simulink model "seminar2part2"  (R2023a)
settings: Solver=VariableStepAuto  StartTime=0.0  StopTime=1  RelTol=1e-3
libraries: spsDiodeLib x6, spsCurrentMeasurementLib x3, spsRMSLib x3, spsVoltageMeasurementLib x2, spsGroundLib x1, eePowerMeasurement x1, spsParallelRLCBranchLib x1, spsTHDLib x1, spsThreePhaseVIMeasurementLib x1, spsThreePhaseSourceLib x1, spspowerguiLib x1
settings Model: Creator=11094  LastModifiedBy=11094
settings DataIOCC: ReturnWorkspaceOutputs=off

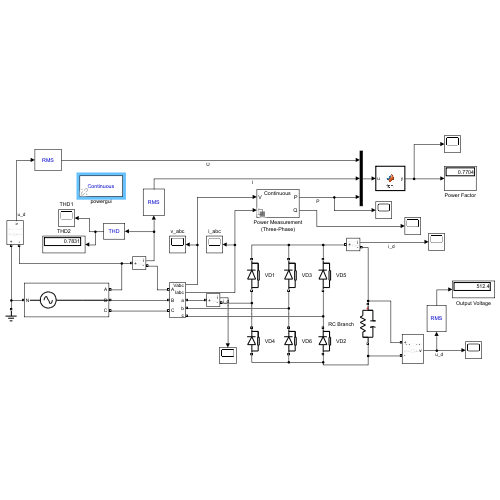
[thumbnail: Simulink's stored preview of the top-level diagram]
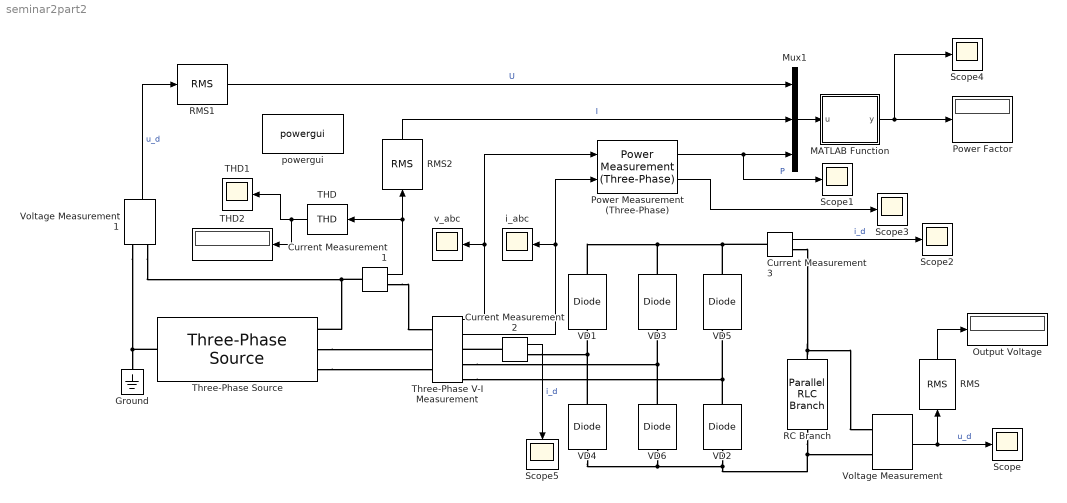
== system seminar2part2 ==
  Current Measurement1 : spsCurrentMeasurementLib/Current Measurement  PhasorSimulation=off  OutputType=Complex  PSBequivalent=0
  Current Measurement2 : spsCurrentMeasurementLib/Current Measurement  PhasorSimulation=off  OutputType=Complex  PSBequivalent=0
  Current Measurement3 : spsCurrentMeasurementLib/Current Measurement  PhasorSimulation=off  OutputType=Complex  PSBequivalent=0
  Ground : spsGroundLib/Ground  LConnTagsString=a
  MATLAB Function : MATLAB Function  TreatAsAtomicUnit=on
  Mux1 : Mux  Inputs=3
  Output Voltage : Display
  Power Factor : Display
  Power Measurement (Three-Phase) : eePowerMeasurement/Power Measurement (Three-Phase)  LabelModeActiveChoice=Continuous  F=50  K=[1]  Seq=Positive  Ts=0
  RC Branch : spsParallelRLCBranchLib/Parallel RLC Branch  LConnTagsString=a  RConnTagsString=__new0  BranchType=RC  Resistance=1  Inductance=1e-3  SetiL0=off  InitialCurrent=0  Capacitance=8e-3  Setx0=off  InitialVoltage=0  Measurements=None
  RMS : spsRMSLib/RMS  TrueRMS=on  Freq=60  RMSInit=120  Ts=0
  RMS1 : spsRMSLib/RMS  TrueRMS=on  Freq=50  RMSInit=120  Ts=0
  RMS2 : spsRMSLib/RMS  TrueRMS=on  Freq=50  RMSInit=120  Ts=0
  Scope{,1..5} (6 alike) : Scope
  THD : spsTHDLib/THD  Freq=50  Ts=0
  THD1 : Scope
  THD2 : Display
  Three-Phase V-I Measurement : spsThreePhaseVIMeasurementLib/Three-Phase V-I Measurement  VoltageMeasurement=phase-to-ground  SetLabelV=off  LabelV=Vabc  Vpu=off  VpuLL=off  CurrentMeasurement=yes  SetLabelI=off  LabelI=Iabc  Ipu=off  Pbase=100e6  Vbase=500e3  OutputType=Complex  PhasorSimulation=off  PSBequivalent=0
  Three-Phase Source : spsThreePhaseSourceLib/Three-Phase Source  InternalConnection=Yn  VoltagePhases=on  Voltage=220  PhaseAngle=0  Voltage_phases=[220 220 220]  PhaseAngles_phases=[0 -120 +120]  Frequency=50  NonIdealSource=on  SpecifyImpedance=off  Resistance=0  Inductance=0  ShortCircuitLevel=100e6  BaseVoltage=25000  XRratio=7  BusType=swing  Pref=10e3  Qref=0  Prefabc=[10e3, 10e3, 10e3]  Qrefabc=[0, 0, 0]  Qmin=-inf  Qmax=inf
  VD{1..6} (6 alike) : spsDiodeLib/Diode  Ron=0.001  Lon=0  Vf=0.8  IC=0  UseSnubber=0  Rs=500  Cs=250e-9  Measurements=off
  Voltage Measurement : spsVoltageMeasurementLib/Voltage Measurement  PhasorSimulation=off  OutputType=Complex  PSBequivalent=0
  Voltage Measurement1 : spsVoltageMeasurementLib/Voltage Measurement  PhasorSimulation=off  OutputType=Complex  PSBequivalent=0
  i_abc : Scope
  powergui : spspowerguiLib/powergui  Priority=1  SimulationMode=Continuous  SampleTime=50e-6  frequency=60  Iterations=50  frequencyindice=50  Pbase=100e6  ErrMax=1e-4  UnitsV=kV  UnitsW=MW  buscounter=0  FunctionMessages=off  echomessages=off  EnableUseOfTLC=off  CurrentSourceSwitches=off  DisableSnubberDevices=off  DisableRonSwitches=off  DisableVfSwitches=off  DisplayEquations=off  AutomaticDiscreteSolvers=off  SolverType=Tustin/Backward Euler (TBE)  Interpol=off  ExternalGateDelay=off  methode=off  Ts=100  x0status=blocks  SPID=on  SwTol=0  HookPort=off  NonlinearTolerance=1e-4  nMaxIteration=100  ContinueOnMaxIteration=off  RestoreLinks=warning  ResistiveCurrentMeasurement=off  Frange=[0:2:500]  Ylog=off  Xlog=on  ShowGrid=off  save=off  variable=ZData  structure=0  ZoomFFT=off  StartTime=0.0  cycles=1  DisplayStyle=1  fundamental=60  FreqAxis=off  MaxFrequency=1000  frequencyindicesteady=1  RmsSteady=1  display=off
  v_abc : Scope
  wires:
  RMS/1 -> Output Voltage/1
  Three-Phase V-I Measurement/1 -> Power Measurement (Three-Phase)/1, v_abc/1
  THD/1 -> THD2/1, THD1/1
  Voltage Measurement/1 -> Scope/1, RMS/1  "u_d"
  Three-Phase V-I Measurement/2 -> i_abc/1, Power Measurement (Three-Phase)/2
  Current Measurement3/1 -> Scope2/1  "i_d"
  Power Measurement (Three-Phase)/1 -> Scope1/1, Mux1/3  "P"
  MATLAB Function/1(y) -> Scope4/1, Power Factor/1
  RMS1/1 -> Mux1/1  "U"
  Mux1/1 -> MATLAB Function/1(u)
  RMS2/1 -> Mux1/2  "I"
  Current Measurement1/1 -> THD/1, RMS2/1
  Voltage Measurement1/1 -> RMS1/1  "u_d"
  Power Measurement (Three-Phase)/2 -> Scope3/1
  Current Measurement2/1 -> Scope5/1  "i_d"
  connections:
  Three-Phase Source/LConn1 -- Voltage Measurement1/LConn1 -- Ground/LConn1
  VD4/RConn1 -- Current Measurement2/RConn1 -- VD1/LConn1
  VD6/LConn1 -- RC Branch/RConn1 -- Voltage Measurement/LConn2 -- VD2/LConn1 -- VD4/LConn1
  RC Branch/LConn1 -- Current Measurement3/RConn1 -- Voltage Measurement/LConn1
  Three-Phase V-I Measurement/RConn3 -- VD5/LConn1 -- VD2/RConn1
  Current Measurement1/LConn1 -- Voltage Measurement1/LConn2 -- Three-Phase Source/RConn1
  Three-Phase V-I Measurement/RConn2 -- VD3/LConn1 -- VD6/RConn1
  Current Measurement1/RConn1 -- Three-Phase V-I Measurement/LConn1
  Three-Phase Source/RConn2 -- Three-Phase V-I Measurement/LConn2
  Three-Phase Source/RConn3 -- Three-Phase V-I Measurement/LConn3
  VD3/RConn1 -- VD1/RConn1 -- VD5/RConn1 -- Current Measurement3/LConn1
  Current Measurement2/LConn1 -- Three-Phase V-I Measurement/RConn1

== matlab function seminar2part2/MATLAB Function ==
  data: u input; y output
function y = fcn(u)

y = u(3)/(3*u(1)*u(2));
